simulink library "tqr"  (R2021b)
settings: Solver=VariableStepAuto  StartTime=0.0  StopTime=10.0  RelTol=1e-3
undefined symbols (not defined in the file or in its folder): ATQR_AltRDCActiveFEDUInc_X_pct, ATQR_AltRDCActiveFEDUInc_Y_enum, ATQR_AltRDCActiveFEDUTs_X_pct, ATQR_AltRDCActiveFEDUTs_Y_enum, ATQR_AltRDCActiveREDUInc_X_pct, ATQR_AltRDCActiveREDUInc_Y_enum, ATQR_AltRDCActiveREDUTs_X_pct, ATQR_AltRDCActiveREDUTs_Y_enum, ATQR_CreepFEDUTqIncSR_X_rpm, ATQR_CreepFEDUTqIncSR_Y_Nm, ATQR_CreepFEDUTs_X_rpm, ATQR_CreepFEDUTs_Y_Nm, ATQR_EcoTqFrIncGain_X_Nm, ATQR_EcoTqFrIncGain_Y_pct, ATQR_EcoTqRrIncGain_X_Nm, ATQR_EcoTqRrIncGain_Y_pct, ATQR_EL1FEDUTqDecSR_Y_Nm, ATQR_EL1FEDUTqIncSR_X_rpm, ATQR_EL1FEDUTqIncSR_Y_pct, ATQR_EL1FEDUTs_X_rpm, ATQR_EL1FEDUTs_Y_Nm, ATQR_EL1REDUTqDecSR_Y_Nm, ATQR_EL1REDUTs_Y_Nm, ATQR_FEDUEL1RegenTs_X_rpm, ATQR_FEDUTIPOutTs_X_rpm, ATQR_FrNegRateLimitIncN_X_rpm, ATQR_FrNegRateLimitIncN_Y_Nm, ATQR_FrPosRateLimitIncN_X_rpm, ATQR_FrPosRateLimitIncN_Y_Nm, ATQR_FShaftSpdTqLimCoe_X_rpm, ATQR_FTimerTqLimCoe_X_s, ATQR_FTqZeroTransUpBoundN_X_rpm, ATQR_NL1FEDUTqDecSR_Y_Nm, ATQR_NL1FEDUTqIncSR_X_rpm, ATQR_NL1FEDUTqIncSR_Y_pct, ATQR_NL1FEDUTs_X_rpm, ATQR_NL1FEDUTs_Y_Nm, ATQR_NL1REDUTqDecSR_Y_Nm, ATQR_NL1REDUTs_Y_Nm, ATQR_NormalTqFrIncGain_X_Nm, ATQR_NormalTqFrIncGain_Y_pct, ATQR_NormalTqRrIncGain_X_Nm, ATQR_NormalTqRrIncGain_Y_pct, ATQR_RrNegRateLimitIncN_X_rpm, ATQR_RrNegRateLimitIncN_Y_Nm, ATQR_RrPosRateLimitIncN_X_rpm, ATQR_RrPosRateLimitIncN_Y_Nm, ATQR_RShaftSpdTqLimCoe_X_rpm, ATQR_RTimerTqLimCoe_X_s, ATQR_SL1FEDUTqDecSR_Y_Nm, ATQR_SL1FEDUTqIncSR_X_rpm, ATQR_SL1FEDUTqIncSR_Y_pct, ATQR_SL1FEDUTs_X_rpm, ATQR_SL1FEDUTs_Y_Nm, ATQR_SL1REDUTqDecSR_Y_Nm, ATQR_SL1REDUTs_Y_Nm, ATQR_SportTqFrIncGain_X_Nm, ATQR_SportTqFrIncGain_Y_pct, ATQR_SportTqRrIncGain_X_Nm, ATQR_SportTqRrIncGain_Y_pct ... (+287)
libraries: hcu_lib x19, simulink x17, $bdroot x3
(part 5 of 10)

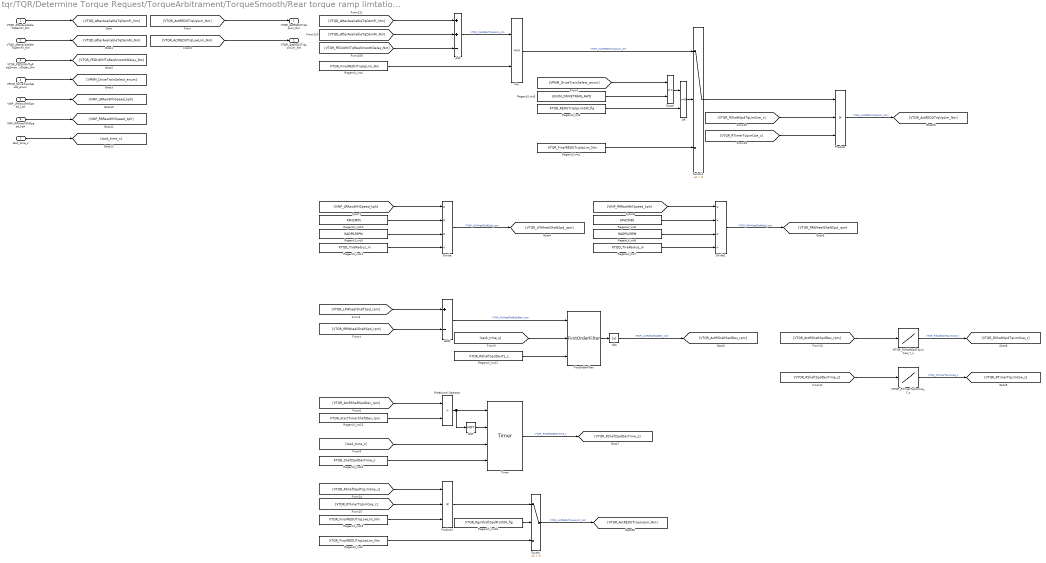
== system tqr/TQR/Determine Torque Request/TorqueArbitrament/TorqueSmooth/Rear torque ramp limtation and determination ==
  VTQD_AfterAvailableTqDemFr_Nm : Inport
  VTQD_AfterAvailableTqDemRr_Nm : Inport  Port=2
  VTQR_FEDUWhlTqReqSmoothDelay_Nm : Inport  Port=3
  VPMM_DriveTrainSelect_enum : Inport  Port=4
  VINP_LRRawWhlSpeed_kph : Inport  Port=5
  VINP_RRRawWhlSpeed_kph : Inport  Port=6
  task_time_s : Inport  Port=7
  Abs : Abs
  Add : Sum  Inputs=++-
  Add1 : Sum  Inputs=+-
  Divide : Product  Inputs=***/
  Divide1 : Product  Inputs=***/
  Equal : RelationalOperator  Operator===  OutDataTypeStr=boolean  RndMeth=Simplest
  FirstOrderFilter : hcu_lib/Basic_Blocks/FirstOrderFilter
  MTQR_RShaftSpdTqLimCoe_Y_c : Lookup_n-D  NumberOfTableDimensions=1  BreakpointsForDimension1=ATQR_RShaftSpdTqLimCoe_X_rpm  Table=MTQR_RShaftSpdTqLimCoe_Y_c  InternalRulePriority=Speed  RndMeth=Simplest  InputSameDT=on
  MTQR_RTimerTqLimCoe_Y_c : Lookup_n-D  NumberOfTableDimensions=1  BreakpointsForDimension1=ATQR_RTimerTqLimCoe_X_s  Table=MTQR_RTimerTqLimCoe_Y_c  InternalRulePriority=Speed  RndMeth=Simplest  InputSameDT=on
  Min : MinMax  Inputs=2
  NOT : Logic  Operator=NOT  AllPortsSameDT=off  OutDataTypeStr=boolean
  OR : Logic  AllPortsSameDT=off  OutDataTypeStr=boolean
  Product : Product  Inputs=3
  Product1 : Product  Inputs=3
  RegenLV_inc1 : Constant  Value=KTQR_FinalREDUTrqUpLim_Nm  OutDataTypeStr=single
  RegenLV_inc10 : Constant  Value=KPH2MPS  OutDataTypeStr=single
  RegenLV_inc11 : Constant  Value=KTQD_TireRadius_m  OutDataTypeStr=single
  RegenLV_inc12 : Constant  Value=KTQR_RShaftSpdDevTs_c  OutDataTypeStr=single
  RegenLV_inc13 : Constant  Value=KTQR_StartTimerShaftDev_rpm  OutDataTypeStr=single
  RegenLV_inc14 : Constant  Value=KTQR_ShaftSpdDevTime_s  OutDataTypeStr=single
  RegenLV_inc15 : Constant  Value=KTQR_FinalREDUTrqLowLim_Nm  OutDataTypeStr=single
  RegenLV_inc16 : Constant  Value=KTQR_RgnShaftSpdProtSW_flg  OutDataTypeStr=single
  RegenLV_inc2 : Constant  Value=KTQR_FinalREDUTrqLowLim_Nm  OutDataTypeStr=single
  RegenLV_inc3 : Constant  Value=KTQR_REDUTrqUpLimSW_flg  OutDataTypeStr=single
  RegenLV_inc4 : Constant  Value=KTQR_FinalREDUTrqUpLim_Nm  OutDataTypeStr=single
  RegenLV_inc5 : Constant  Value=ENUM_DRIVETRAIN_AWD  OutDataTypeStr=single
  RegenLV_inc6 : Constant  Value=KPH2MPS  OutDataTypeStr=single
  RegenLV_inc7 : Constant  Value=KTQD_TireRadius_m  OutDataTypeStr=single
  RegenLV_inc8 : Constant  Value=RADPS2RPM  OutDataTypeStr=single
  RegenLV_inc9 : Constant  Value=RADPS2RPM  OutDataTypeStr=single
  Relational Operator : RelationalOperator  Operator=>  OutDataTypeStr=boolean  RndMeth=Simplest
  Switch : Switch  Criteria=u2 > Threshold
  Switch1 : Switch  Criteria=u2 > Threshold
  Timer : hcu_lib/Basic_Blocks/Timer
  VTQR_ActREDUTrqUpLim_Nm : Outport
  VTQR_ActREDUTrqLowLim_Nm : Outport  Port=2
  wires:
  Add/1 -> Min/1  "VTQR_CalREDUTrqUpLim_Nm"
  RegenLV_inc4/1 -> Min/2
  [VTQR_FEDUWhlTqReqSmoothDelay_Nm] -> Add/3
  Min/1 -> Switch1/1  "VTQR_CoorREDUTrqUpLim_Nm"
  [VTQD_AfterAvailableTqDemFr_Nm] -> Add/1
  [VTQD_AfterAvailableTqDemRr_Nm] -> Add/2
  RegenLV_inc1/1 -> Switch1/3
  VTQD_AfterAvailableTqDemFr_Nm/1 -> [VTQD_AfterAvailableTqDemFr_Nm]
  VTQD_AfterAvailableTqDemRr_Nm/1 -> [VTQD_AfterAvailableTqDemRr_Nm]
  VTQR_FEDUWhlTqReqSmoothDelay_Nm/1 -> [VTQR_FEDUWhlTqReqSmoothDelay_Nm]
  VPMM_DriveTrainSelect_enum/1 -> [VPMM_DriveTrainSelect_enum]
  [VTQR_ActREDUTrqUpLim_Nm] -> VTQR_ActREDUTrqUpLim_Nm/1
  [VTQR_ActREDUTrqLowLim_Nm] -> VTQR_ActREDUTrqLowLim_Nm/1
  OR/1 -> Switch1/2
  Equal/1 -> OR/1
  RegenLV_inc5/1 -> Equal/2
  [VPMM_DriveTrainSelect_enum] -> Equal/1
  RegenLV_inc3/1 -> OR/2
  RegenLV_inc10/1 -> Divide/2
  RegenLV_inc9/1 -> Divide/3
  RegenLV_inc11/1 -> Divide/4
  Divide/1 -> [VTQR_LFWheelShaftSpd_rpm]  "VTQR_LRWheelShaftSpd_rpm"
  Divide1/1 -> [VTQR_RRWheelShaftSpd_rpm]  "VTQR_RRWheelShaftSpd_rpm"
  RegenLV_inc7/1 -> Divide1/4
  RegenLV_inc8/1 -> Divide1/3
  RegenLV_inc6/1 -> Divide1/2
  [VINP_RRRawWhlSpeed_kph] -> Divide1/1
  Add1/1 -> FirstOrderFilter/1  "VTQR_RWheelShaftSpdDev_rpm"
  [task_time_s] -> FirstOrderFilter/2
  [VTQR_RRWheelShaftSpd_rpm] -> Add1/2
  RegenLV_inc12/1 -> FirstOrderFilter/3
  FirstOrderFilter/1 -> Abs/1
  Abs/1 -> [VTQR_ActRShaftSpdDev_rpm]  "VTQR_ActRShaftSpdDev_rpm"
  [VTQR_ActRShaftSpdDev_rpm] -> Relational Operator/1
  [VTQR_LFWheelShaftSpd_rpm] -> Add1/1
  RegenLV_inc13/1 -> Relational Operator/2
  Relational Operator/1 -> Timer/1, NOT/1
  NOT/1 -> Timer/2
  [task_time_s] -> Timer/3
  RegenLV_inc14/1 -> Timer/4
  Timer/1 -> [VTQR_RShaftSpdDevTime_s]  "VTQR_RShaftSpdDevTime_s"
  [VTQR_ActRShaftSpdDev_rpm] -> MTQR_RShaftSpdTqLimCoe_Y_c/1
  MTQR_RShaftSpdTqLimCoe_Y_c/1 -> [VTQR_RShaftSpdTqLimCoe_c]  "VTQR_RShaftSpdTqLimCoe_c"
  MTQR_RTimerTqLimCoe_Y_c/1 -> [VTQR_RTimerTqLimCoe_c]  "VTQR_RTimerTqLimCoe_c"
  [VTQR_RShaftSpdDevTime_s] -> MTQR_RTimerTqLimCoe_Y_c/1
  Product/1 -> [VTQR_ActREDUTrqUpLim_Nm]  "VTQR_ActREDUTrqUpLim_Nm"
  Switch1/1 -> Product/1
  [VTQR_RShaftSpdTqLimCoe_c] -> Product/2
  [VTQR_RTimerTqLimCoe_c] -> Product/3
  task_time_s/1 -> [task_time_s]
  VINP_RRRawWhlSpeed_kph/1 -> [VINP_RRRawWhlSpeed_kph]
  VINP_LRRawWhlSpeed_kph/1 -> [VINP_LRRawWhlSpeed_kph]
  [VINP_LRRawWhlSpeed_kph] -> Divide/1
  Switch/1 -> [VTQR_ActREDUTrqLowLim_Nm]  "VTQR_ActREDUTrqLowLim_Nm"
  RegenLV_inc2/1 -> Switch/3
  Product1/1 -> Switch/1
  RegenLV_inc15/1 -> Product1/3
  [VTQR_RTimerTqLimCoe_c] -> Product1/2
  [VTQR_RShaftSpdTqLimCoe_c] -> Product1/1
  RegenLV_inc16/1 -> Switch/2

== system tqr/TQR/Determine Torque Request/TorqueArbitrament/TorqueSmooth/Rear wheel first order filter input torque command determination ==
  VTQR_RrTqZeroTrans_enum : Inport
  VTQR_RrTqZeroTransUpBound_Nm : Inport  Port=2
  VTQR_RrTqZeroTransLowBound_Nm : Inport  Port=3
  VTQD_AfterAvailableTqDemRr_Nm : Inport  Port=4
  VTQR_RrFirstOrderOutTqDelay_Nm : Inport  Port=5
  VTQR_RrGearChange_flg : Inport  Port=6
  VTQR_RampTqCMDGain_c : Inport  Port=7
  AND : Logic  AllPortsSameDT=off  OutDataTypeStr=boolean
  Constant1 : Constant  Value=ZERO_FLOAT
  Constant2 : Constant  Value=KTQR_GearChangeTqSW_flg
  Constant3 : Constant  Value=ENUM_TQZEROTRANS_NOZEROTRANS
  Constant4 : Constant  Value=KTQR_NewRampArchSW_flg
  Constant5 : Constant  Value=ONE_FLOAT
  Product : Product
  Relational Operator : RelationalOperator  Operator===  OutDataTypeStr=boolean  RndMeth=Simplest
  Relational Operator1 : RelationalOperator  OutDataTypeStr=boolean  RndMeth=Simplest
  Relational Operator2 : RelationalOperator  Operator=<=  OutDataTypeStr=boolean  RndMeth=Simplest
  Switch : Switch  Criteria=u2 ~= 0
  Switch1 : Switch  Criteria=u2 ~= 0
  Switch2 : Switch  Criteria=u2 ~= 0
  Switch3 : Switch  Criteria=u2 > Threshold
  Switch4 : Switch  Criteria=u2 > Threshold
  VTQR_RrFirstOrderInpTq_Nm : Outport
  wires:
  Switch3/1 -> VTQR_RrFirstOrderInpTq_Nm/1  "VTQR_RrFirstOrderInpTq_Nm"
  [VTQR_RrTqZeroTransUpBound_Nm] -> Switch1/1
  [VTQR_RrTqZeroTransUpBound_Nm] -> Relational Operator1/2
  [VTQR_RrFirstOrderOutTqDelay_Nm] -> Relational Operator1/1
  Relational Operator1/1 -> Switch1/2
  Switch1/1 -> Switch/3
  Relational Operator/1 -> Switch/2
  Constant3/1 -> Relational Operator/2
  [VTQR_RrTqZeroTrans_enum] -> Relational Operator/1
  Relational Operator2/1 -> Switch2/2
  [VTQR_RrActRampTqDem_Nm] -> Switch2/3
  [VTQR_RrTqZeroTransLowBound_Nm] -> Switch2/1
  [VTQR_RrFirstOrderOutTqDelay_Nm] -> Relational Operator2/1
  [VTQR_RrTqZeroTransLowBound_Nm] -> Relational Operator2/2
  Switch2/1 -> Switch1/3
  VTQR_RrTqZeroTransUpBound_Nm/1 -> [VTQR_RrTqZeroTransUpBound_Nm]
  VTQR_RrTqZeroTransLowBound_Nm/1 -> [VTQR_RrTqZeroTransLowBound_Nm]
  VTQR_RrFirstOrderOutTqDelay_Nm/1 -> [VTQR_RrFirstOrderOutTqDelay_Nm]
  VTQR_RrGearChange_flg/1 -> [VTQR_RrGearChange_flg]
  VTQR_RrTqZeroTrans_enum/1 -> [VTQR_RrTqZeroTrans_enum]
  VTQD_AfterAvailableTqDemRr_Nm/1 -> [VTQD_AfterAvailableTqDemRr_Nm]
  Constant2/1 -> AND/2
  Constant1/1 -> Switch3/1
  [VTQR_RrGearChange_flg] -> AND/1
  AND/1 -> Switch3/2
  Switch/1 -> Switch3/3
  VTQR_RampTqCMDGain_c/1 -> [VTQR_RampTqCMDGain_c]
  Product/1 -> [VTQR_RrActRampTqDem_Nm]  "VTQR_RrActRampTqDem_Nm"
  Constant4/1 -> Switch4/2
  Switch4/1 -> Product/2
  Constant5/1 -> Switch4/3
  [VTQR_RampTqCMDGain_c] -> Switch4/1
  [VTQR_RrActRampTqDem_Nm] -> Switch/1
  [VTQD_AfterAvailableTqDemRr_Nm] -> Product/1

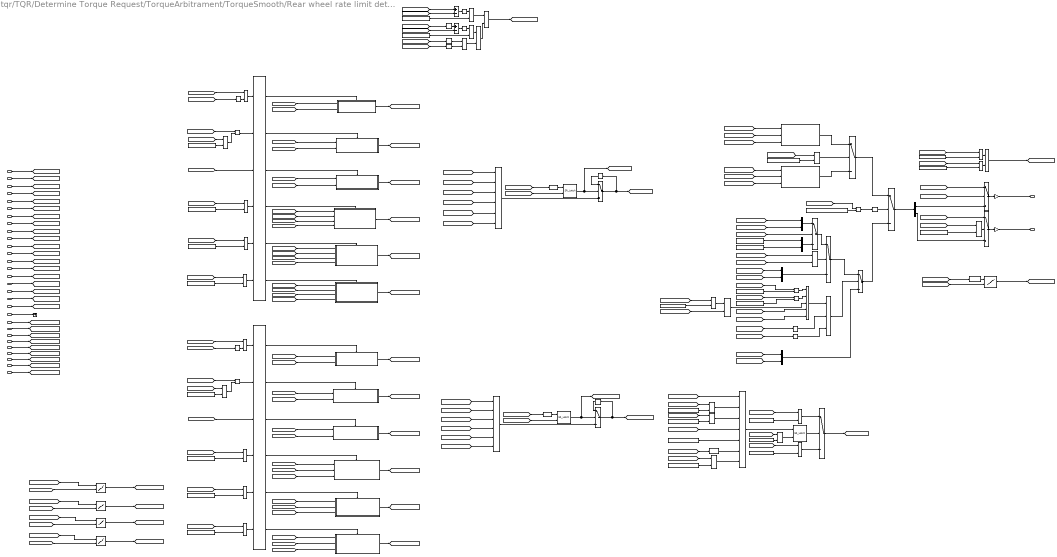
== system tqr/TQR/Determine Torque Request/TorqueArbitrament/TorqueSmooth/Rear wheel rate limit determination ==
  VTQR_RrTqZeroTrans_enum : Inport
  VTQD_TqSourceRr_enum : Inport  Port=2
  VTQD_TqTargetShaftSpd_rpm : Inport  Port=3
  VTQD_LimpHomeAct_flg : Inport  Port=4
  VTQR_EVDriveMode_enum : Inport  Port=5
  VDHP_ActAPSPosn_pct : Inport  Port=6
  VTQR_REDUWhlTqReqSmoothDelay_Nm : Inport  Port=7
  VTQD_EVDriveModeValid_flg : Inport  Port=8
  VTQD_RegenMode_enum : Inport  Port=9
  VVMC_ACCPedalOvrd_flg : Inport  Port=10
  VVMC_CCPedalOvrd_flg : Inport  Port=11
  VTQD_CreepPrLoadEnable_flg : Inport  Port=12
  VTQD_RegenTqLimitEn_flg : Inport  Port=13
  VTQD_RDCActive_enum : Inport  Port=14
  VTQD_PreLoadPreEn_flg : Inport  Port=15
  VTQR_NoABSREDUWhlTqReq_Nm : Inport  Port=16
  VTQR_RampREDUWhlTqReq_Nm : Inport  Port=17
  VTQR_RrFirstOrderInpTq_Nm : Inport  Port=18
  VVMC_ActMaxSlideRate_pct : Inport  Port=19
  VTQD_PedAccTqEn_flg : Inport  Port=20
  VVMC_MSAWhlTqActive_flg : Inport  Port=21
  VINP_ACCVehHoldReq_flg : Inport  Port=22
  VINP_GRADE_Deg : Inport  Port=23
  VTQD_VehActSpd_kph : Inport  Port=24
  VVMC_ADASActive_flg : Inport  Port=25
  VPMM_DriveTrainSelect_enum : Inport  Port=26
  VINP_RrPTCSActive_flg : Inport  Port=27
  VINP_IVISnowModeCmd_flg : Inport  Port=28
  VINP_VehicleType_enum : Inport  Port=29
  AND{,2..4} (4 alike) : Logic  AllPortsSameDT=off  OutDataTypeStr=boolean
  AND1 : Logic  Inputs=3  AllPortsSameDT=off  OutDataTypeStr=boolean
  AND5 : Logic  Inputs=7  AllPortsSameDT=off  OutDataTypeStr=boolean
  Abs : Abs
  Abs4 : Abs
  Add : Sum  Inputs=+-
  Add1 : Sum  Inputs=+-
  Constant : Constant  Value=KTQR_ACCHoldPdovrdGrade_Deg
  Constant1 : Constant  Value=ENUM_TQZEROTRANS_NOZEROTRANS
  Constant10 : Constant  Value=ENUM_TQSOURCE_MSA
  Constant11 : Constant  Value=KTQR_ACCHoldPdovrdVeh_kph
  Constant12 : Constant  Value=KTQR_ARegenLatchEnTq_Nm
  Constant13 : Constant  Value=KTQR_ACCHoldPdovrdSW_flg
  Constant14 : Constant  Value=ENUM_DRIVETRAIN_RWD
  Constant15 : Constant  Value=KTQR_ACCHoldPdovrdInc_Nm
  Constant16 : Constant  Value=KTQR_ACCHoldPdovrdInc_Nm
  Constant17 : Constant  Value=ZERO_FLOAT
  Constant18 : Constant  Value=ENUM_VEHICLETYPE_D31L24
  Constant19 : Constant  Value=ENUM_VEHICLETYPE_D31L24
  Constant2 : Constant  Value=KTQR_DriveModeChangeTq_Nm
  Constant22 : Constant  Value=ENUM_DRIVEMODE_ECO
  Constant23 : Constant  Value=ENUM_DRIVEMODE_NRM
  Constant24 : Constant  Value=ENUM_DRIVEMODE_SPORT
  Constant26 : Constant  Value=ENUM_DRIVEMODE_ECO
  Constant27 : Constant  Value=ENUM_DRIVEMODE_NRM
  Constant28 : Constant  Value=ENUM_DRIVEMODE_SPORT
  Constant3 : Constant  Value=ENUM_TQSOURCE_CC
  Constant34 : Constant  Value=ENUM_TQSOURCE_ADAS
  Constant4 : Constant  Value=ENUM_TQZEROTRANS_POSITIVE
  Constant5 : Constant  Value=ENUM_RDCACTSTA_NOREQUEST
  Constant6 : Constant  Value=KTQR_RegenTqLimitDecSW_flg
  Constant7 : Constant  Value=KTQR_PreLoadTqIncSR_Nm
  Constant8 : Constant  Value=KTQR_DriveModeCMDTqDev_Nm
  Constant9 : Constant  Value=KTQR_PreLoadTqDecSR_Nm
  Data Type Conversion : DataTypeConversion  OutDataTypeStr=single
  Delay{,1..4} (5 alike) : Delay  DelayLength=1
  Demux : Demux  Outputs=2
  Detect Change : simulink/Logic and Bit Operations/Detect Change  vinit=0  OutDataTypeStr=boolean
  Detect Change1 : simulink/Logic and Bit Operations/Detect Change  vinit=0  OutDataTypeStr=boolean
  Detect Increase : simulink/Logic and Bit Operations/Detect Increase  vinit=0.0  OutDataTypeStr=boolean
  Equal : RelationalOperator  OutDataTypeStr=boolean  RndMeth=Simplest
  Equal1 : RelationalOperator  Operator=<=  OutDataTypeStr=boolean  RndMeth=Simplest
  Equal2 : RelationalOperator  Operator=~=  OutDataTypeStr=boolean  RndMeth=Simplest
  Equal{3,20..21,23..25,27} (7 alike) : RelationalOperator  Operator===  OutDataTypeStr=boolean  RndMeth=Simplest
  Equal4 : RelationalOperator  OutDataTypeStr=boolean  RndMeth=Simplest
  Equal5 : RelationalOperator  Operator=~=  OutDataTypeStr=boolean  RndMeth=Simplest
  Equal6 : RelationalOperator  Operator=~=  OutDataTypeStr=boolean  RndMeth=Simplest
  Gain : Gain
  Gain1 : Gain
  If : If  NumInputs=6  IfExpression=u1~= 0  ElseIfExpressions=u2 ~= 0, u3 ~= 0,u4 ~= 0,u5 ~= 0
  If1 : If  NumInputs=6  IfExpression=u1~= 0  ElseIfExpressions=u2 ~= 0, u3 ~= 0,u4 ~= 0,u5 ~= 0
  Logical Operator : Logic  AllPortsSameDT=off  OutDataTypeStr=boolean
  Logical Operator1 : Logic  AllPortsSameDT=off  OutDataTypeStr=boolean
  Logical Operator10 : Logic  Operator=OR  AllPortsSameDT=off  OutDataTypeStr=boolean
  Logical Operator11 : Logic  Operator=NOT  AllPortsSameDT=off  OutDataTypeStr=boolean
  Logical Operator12 : Logic  Operator=OR  AllPortsSameDT=off  OutDataTypeStr=boolean
  Logical Operator13 : Logic  Operator=NOT  AllPortsSameDT=off  OutDataTypeStr=boolean
  Logical Operator14 : Logic  Operator=OR  Inputs=5  AllPortsSameDT=off  OutDataTypeStr=boolean
  Logical Operator7 : Logic  Operator=NOT  AllPortsSameDT=off  OutDataTypeStr=boolean
  MTQR_AltRDCActiveREDUInc_Z_Nm : Lookup_n-D  BreakpointsForDimension1=ATQR_AltRDCActiveREDUInc_Y_enum  BreakpointsForDimension2=ATQR_AltRDCActiveREDUInc_X_pct  Table=MTQR_AltRDCActiveREDUInc_Z_Nm  TableDataTypeStr=Inherit: Inherit from 'Table data'  ExtrapMethod=Clip  InternalRulePriority=Speed  RndMeth=Simplest  InputSameDT=on
      settings: InputPortMap=u0,u1
  MTQR_CreepREDUTqDecSR_Z_Nm : Lookup_n-D  BreakpointsForDimension1=ATQR_CreepFEDUTqIncSR_Y_Nm  BreakpointsForDimension2=ATQR_CreepFEDUTqIncSR_X_rpm  Table=MTQR_CreepREDUTqDecSR_Z_Nm  ExtrapMethod=Clip  InternalRulePriority=Speed  RndMeth=Simplest  InputSameDT=on
      settings: InputPortMap=u0,u1
  MTQR_CreepREDUTqIncSR_Z_Nm : Lookup_n-D  BreakpointsForDimension1=ATQR_CreepFEDUTqIncSR_Y_Nm  BreakpointsForDimension2=ATQR_CreepFEDUTqIncSR_X_rpm  Table=MTQR_CreepREDUTqIncSR_Z_Nm  ExtrapMethod=Clip  InternalRulePriority=Speed  RndMeth=Simplest  InputSameDT=on
      settings: InputPortMap=u0,u1
  MTQR_VMCREDUTqDecSR_Z_Nm : Lookup_n-D  BreakpointsForDimension1=ATQR_VMCREDUTqIncSR_Y_Nm  BreakpointsForDimension2=ATQR_VMCFEDUTqIncSR_X_rpm  Table=MTQR_VMCREDUTqDecSR_Z_Nm  ExtrapMethod=Clip  InternalRulePriority=Speed  RndMeth=Simplest  InputSameDT=on
      settings: InputPortMap=u0,u1
  MTQR_VMCREDUTqIncSR_Z_Nm : Lookup_n-D  BreakpointsForDimension1=ATQR_VMCREDUTqIncSR_Y_Nm  BreakpointsForDimension2=ATQR_VMCFEDUTqIncSR_X_rpm  Table=MTQR_VMCREDUTqIncSR_Z_Nm  ExtrapMethod=Clip  InternalRulePriority=Speed  RndMeth=Simplest  InputSameDT=on
      settings: InputPortMap=u0,u1
  Max : MinMax  Function=max  Inputs=2
  Max1 : MinMax  Function=max  Inputs=2
  Merge4 : Merge  Inputs=6
  Merge5 : Merge  Inputs=6
  Mux{1..4} (4 alike) : Mux  Inputs=2
  NOT : Logic  Operator=NOT  AllPortsSameDT=off  OutDataTypeStr=boolean
  NOT1 : Logic  Operator=NOT  AllPortsSameDT=off  OutDataTypeStr=boolean
  Negative Rate limit Determination : Subsystem  TreatAsAtomicUnit=on
  OR : Logic  Operator=OR  AllPortsSameDT=off  OutDataTypeStr=boolean
  OR2 : Logic  Operator=OR  AllPortsSameDT=off  OutDataTypeStr=boolean
  OR3 : Logic  Operator=OR  AllPortsSameDT=off  OutDataTypeStr=boolean
  Positive Rate limit Determination : Subsystem  TreatAsAtomicUnit=on
  Relational Operator{,1,3..4,7} (5 alike) : RelationalOperator  Operator===  OutDataTypeStr=boolean  RndMeth=Simplest
  Relational Operator2 : RelationalOperator  Operator=<=  OutDataTypeStr=boolean  RndMeth=Simplest
  Relational Operator5 : RelationalOperator  Operator=<  OutDataTypeStr=boolean  RndMeth=Simplest
  Relational Operator6 : RelationalOperator  OutDataTypeStr=boolean  RndMeth=Simplest
  SR_Latch1 : hcu_lib/Basic_Blocks/SR_Latch
  SR_Latch2 : hcu_lib/Basic_Blocks/SR_Latch
  SR_Latch3 : hcu_lib/Basic_Blocks/SR_Latch
  Switch{,4..7} (5 alike) : Switch  Criteria=u2 > Threshold
  Switch1 : Switch  Criteria=u2 ~= 0  Threshold=0.5
  Switch13 : Switch  Criteria=u2 ~= 0
  Switch2 : Switch  Criteria=u2 ~= 0
  Switch3 : Switch  Criteria=u2 ~= 0  Threshold=0.5
  Switch8 : Switch  Criteria=u2 ~= 0
  Terminator : Terminator
  VTQR_ECOREDURateLimitDec_Nm : Subsystem  AncestorBlock=tqr/TQR/Determine Torque Request/TorqueArbitrament/TorqueSmooth/Front wheel rate limit determination/VTQR_ECOFEDURateLimitDec_Nm  TreatAsAtomicUnit=on
  VTQR_ECOREDURateLimitInc_Nm : Subsystem  TreatAsAtomicUnit=on
  VTQR_LHMREDURateLimitDec_Nm : Subsystem  AncestorBlock=tqr/TQR/Determine Torque Request/TorqueArbitrament/TorqueSmooth/VTQR_LHMREDURateLimitDec_Nm  TreatAsAtomicUnit=on
  VTQR_LHMREDURateLimitInc_Nm : Subsystem  TreatAsAtomicUnit=on
  VTQR_NORMALREDURateLimitDec_Nm : Subsystem  AncestorBlock=tqr/TQR/Determine Torque Request/TorqueArbitrament/TorqueSmooth/Rear wheel rate limit determination/VTQR_ECOFEDURateLimitDec_Nm  TreatAsAtomicUnit=on
  VTQR_NORMALREDURateLimitInc_Nm : Subsystem  TreatAsAtomicUnit=on
  VTQR_SNOWREDURateLimitDec_Nm : Subsystem  TreatAsAtomicUnit=on
  VTQR_SNOWREDURateLimitInc_Nm : Subsystem  TreatAsAtomicUnit=on
  VTQR_SPORTREDURateLimitDec_Nm : Subsystem  AncestorBlock=tqr/TQR/Determine Torque Request/TorqueArbitrament/TorqueSmooth/Rear wheel rate limit determination/VTQR_ECOFEDURateLimitDec_Nm  TreatAsAtomicUnit=on
  VTQR_SPORTREDURateLimitInc_Nm : Subsystem  TreatAsAtomicUnit=on
  VTQR_TCSREDURateLimitDec_Nm : Subsystem  TreatAsAtomicUnit=on
  VTQR_TCSREDURateLimitInc_Nm : Subsystem  TreatAsAtomicUnit=on
  VTQR_RrRateLimitInc_Nm : Outport
  VTQR_RrRateLimitDec_Nm : Outport  Port=2
  wires:
  VTQD_TqTargetShaftSpd_rpm/1 -> [VTQD_TqTargetShaftSpd_rpm]
  Gain1/1 -> VTQR_RrRateLimitDec_Nm/1  "VTQR_RrRateLimitDec_Nm"
  Gain/1 -> VTQR_RrRateLimitInc_Nm/1  "VTQR_RrRateLimitInc_Nm"
  [VTQR_REDURateLimitDec_Nm] -> Mux4/2
  [VTQR_REDURateLimitInc_Nm] -> Mux4/1
  [VTQR_VMCREDUTqDecSR_Nm] -> Mux3/2
  [VTQR_VMCREDUTqIncSR_Nm] -> Mux3/1
  Positive Rate limit Determination/1(VTQR_PosRateLimit_mux) -> Switch1/1
  Negative Rate limit Determination/1(VTQR_NegRateLimit_mux) -> Switch1/3
  Switch3/1 -> Demux/1
  Switch1/1 -> Switch3/1
  Constant4/1 -> Relational Operator1/2
  Relational Operator1/1 -> Switch1/2
  [VTQR_RrTqZeroTrans_enum] -> Relational Operator1/1
  [VTQR_RrTqZeroTrans_enum] -> Relational Operator/1
  Constant1/1 -> Relational Operator/2
  Relational Operator/1 -> Logical Operator7/1
  Logical Operator7/1 -> Switch3/2
  Switch13/1 -> Switch3/3
  Mux4/1 -> Switch13/3
  AND1/1 -> Switch13/2
  VTQD_TqSourceRr_enum/1 -> [VTQD_TqSourceRr_enum]
  VTQR_RrTqZeroTrans_enum/1 -> [VTQR_RrTqZeroTrans_enum]
  MTQR_VMCREDUTqIncSR_Z_Nm/1 -> [VTQR_VMCREDUTqIncSR_Nm]  "VTQR_VMCREDUTqIncSR_Nm"
  Constant27/1 -> Equal25/2
  [VDHP_ActAPSPosn_pct] -> VTQR_LHMREDURateLimitInc_Nm/1(VDHP_ActAPSPosn_pct)
  [VTQD_LimpHomeAct_flg] -> Logical Operator12/1
  Constant22/1 -> Equal20/2
  MTQR_VMCREDUTqDecSR_Z_Nm/1 -> [VTQR_VMCREDUTqDecSR_Nm]  "VTQR_VMCREDUTqDecSR_Nm"
  [VTQR_EVDriveMode_enum] -> Equal27/1
  Constant28/1 -> Equal27/2
  [VTQR_EVDriveMode_enum] -> Equal25/1
  [VTQD_EVDriveModeValid_flg] -> Logical Operator11/1
  Logical Operator10/1 -> If/1
  Constant24/1 -> Equal23/2
  [VTQD_LimpHomeAct_flg] -> Logical Operator10/1
  Logical Operator11/1 -> Logical Operator10/2
  [VTQR_EVDriveMode_enum] -> Equal20/1
  VTQR_LHMREDURateLimitDec_Nm/1(VTQR_LHMREDURateLimitDec_Nm) -> [VTQR_LHMREDURateLimitDec_Nm]
  [VTQR_REDUWhlTqReqSmoothDelay_Nm] -> VTQR_ECOREDURateLimitDec_Nm/1(VTQR_REDUWhlTqReqSmoothDelay_Nm)
  [VTQD_TqTargetShaftSpd_rpm] -> VTQR_NORMALREDURateLimitDec_Nm/2(VTQD_TqTargetShaftSpd_rpm)  "VTQD_TqTargetShaftSpd_rpm"
  [VTQR_REDUWhlTqReqSmoothDelay_Nm] -> VTQR_LHMREDURateLimitDec_Nm/1(VTQR_REDUWhlTqReqSmooth_Nm)
  [VTQD_TqTargetShaftSpd_rpm] -> VTQR_LHMREDURateLimitDec_Nm/2(VTQD_TqTargetShaftSpd_rpm)  "VTQD_TqTargetShaftSpd_rpm"
  [VTQR_REDUWhlTqReqSmoothDelay_Nm] -> VTQR_NORMALREDURateLimitDec_Nm/1(VTQR_REDUWhlTqReqSmoothDelay_Nm)
  [VTQR_REDUWhlTqReqSmoothDelay_Nm] -> VTQR_SPORTREDURateLimitDec_Nm/1(VTQR_REDUWhlTqReqSmoothDelay_Nm)
  [VTQD_TqTargetShaftSpd_rpm] -> VTQR_LHMREDURateLimitInc_Nm/2(VTQD_TqTargetShaftSpd_rpm)  "VTQD_TqTargetShaftSpd_rpm"
  [VTQD_TqTargetShaftSpd_rpm] -> VTQR_ECOREDURateLimitDec_Nm/2(VTQD_TqTargetShaftSpd_rpm)  "VTQD_TqTargetShaftSpd_rpm"
  [VTQD_TqTargetShaftSpd_rpm] -> VTQR_SPORTREDURateLimitDec_Nm/2(VTQD_TqTargetShaftSpd_rpm)  "VTQD_TqTargetShaftSpd_rpm"
  Constant23/1 -> Equal21/2
  [VTQD_EVDriveModeValid_flg] -> Logical Operator13/1
  [VTQR_EVDriveMode_enum] -> Equal23/1
  Logical Operator13/1 -> Logical Operator12/2
  Constant26/1 -> Equal24/2
  [VTQR_EVDriveMode_enum] -> Equal24/1
  [VTQR_EVDriveMode_enum] -> Equal21/1
  VTQD_LimpHomeAct_flg/1 -> [VTQD_LimpHomeAct_flg]
  VTQR_EVDriveMode_enum/1 -> [VTQR_EVDriveMode_enum]
  VDHP_ActAPSPosn_pct/1 -> [VDHP_ActAPSPosn_pct]
  VTQR_REDUWhlTqReqSmoothDelay_Nm/1 -> [VTQR_REDUWhlTqReqSmoothDelay_Nm]
  VTQD_EVDriveModeValid_flg/1 -> [VTQD_EVDriveModeValid_flg]
  Switch/1 -> Gain/1
  VTQD_RegenMode_enum/1 -> [VTQD_RegenMode_enum]
  [VTQD_RegenMode_enum] -> VTQR_NORMALREDURateLimitDec_Nm/3(VTQD_RegenMode_enum)
  [VTQD_RegenMode_enum] -> VTQR_ECOREDURateLimitDec_Nm/3(VTQD_RegenMode_enum)
  [VTQD_RegenMode_enum] -> VTQR_SPORTREDURateLimitDec_Nm/3(VTQD_RegenMode_enum)
  [VTQD_TqTargetShaftSpd_rpm] -> MTQR_VMCREDUTqIncSR_Z_Nm/2
  [VTQR_REDUWhlTqReqSmoothDelay_Nm] -> MTQR_VMCREDUTqIncSR_Z_Nm/1
  [VTQD_TqTargetShaftSpd_rpm] -> MTQR_VMCREDUTqDecSR_Z_Nm/2
  [VTQR_REDUWhlTqReqSmoothDelay_Nm] -> MTQR_VMCREDUTqDecSR_Z_Nm/1
  VVMC_ACCPedalOvrd_flg/1 -> [VVMC_ACCPedalOvrd_flg]
  VVMC_CCPedalOvrd_flg/1 -> [VVMC_CCPedalOvrd_flg]
  [VTQD_TqSourceRr_enum] -> Relational Operator4/1
  [VTQD_TqSourceRr_enum] -> Relational Operator3/1
  Constant3/1 -> Relational Operator3/2
  Constant34/1 -> Relational Operator4/2
  NOT/1 -> AND1/2
  [VVMC_ACCPedalOvrd_flg] -> NOT/1
  [VVMC_CCPedalOvrd_flg] -> NOT1/1
  NOT1/1 -> AND1/3
  Logical Operator14/1 -> AND1/1
  Relational Operator3/1 -> Logical Operator14/1
  Relational Operator4/1 -> Logical Operator14/2
  [VTQD_TqTargetShaftSpd_rpm] -> Positive Rate limit Determination/1(VTQD_TqTargetShaftSpd_rpm)
  [VTQD_TqTargetShaftSpd_rpm] -> Negative Rate limit Determination/1(VTQD_TqTargetShaftSpd_rpm)
  [VTQR_REDUWhlTqReqSmoothDelay_Nm] -> Positive Rate limit Determination/2(VTQR_REDUWhlTqReqSmoothDelay_Nm)
  [VTQR_EVDriveMode_enum] -> Positive Rate limit Determination/3(VTQR_EVDriveMode_enum)
  [VTQR_REDUWhlTqReqSmoothDelay_Nm] -> Negative Rate limit Determination/2(VTQR_REDUWhlTqReqSmoothDelay_Nm)
  [VTQR_EVDriveMode_enum] -> Negative Rate limit Determination/3(VTQR_EVDriveMode_enum)
  MTQR_CreepREDUTqDecSR_Z_Nm/1 -> [VTQR_CreepREDUTqDecSR_Nm]  "VTQR_CreepREDUTqDecSR_Nm"
  [VTQD_TqTargetShaftSpd_rpm] -> MTQR_CreepREDUTqDecSR_Z_Nm/2
  [VTQD_TqTargetShaftSpd_rpm] -> MTQR_CreepREDUTqIncSR_Z_Nm/2
  MTQR_CreepREDUTqIncSR_Z_Nm/1 -> [VTQR_CreepREDUTqIncSR_Nm]  "VTQR_CreepREDUTqIncSR_Nm"
  [VTQR_REDUWhlTqReqSmoothDelay_Nm] -> MTQR_CreepREDUTqIncSR_Z_Nm/1
  [VTQR_REDUWhlTqReqSmoothDelay_Nm] -> MTQR_CreepREDUTqDecSR_Z_Nm/1
  [VTQD_CreepPrLoadEnable_flg] -> Logical Operator14/4
  [VTQD_PreLoadPreEn_flg] -> Logical Operator14/5
  [VTQD_PreLoadPreEn_flg] -> OR/2
  [VTQD_CreepPrLoadEnable_flg] -> OR/1
  [VTQR_CreepREDUTqIncSR_Nm] -> Mux1/1
  OR/1 -> Switch2/2
  [VTQR_CreepREDUTqDecSR_Nm] -> Mux1/2
  Mux3/1 -> Switch2/3
  Switch2/1 -> Switch13/1
  [VTQR_RrRDCActRateLimitInc_flg] -> Switch/2
  Demux/1 -> Switch/3
  VTQD_CreepPrLoadEnable_flg/1 -> [VTQD_CreepPrLoadEnable_flg]
  VTQD_PreLoadPreEn_flg/1 -> [VTQD_PreLoadPreEn_flg]
  VTQD_RDCActive_enum/1 -> [VTQD_RDCActive_enum]
  VTQR_NoABSREDUWhlTqReq_Nm/1 -> [VTQR_NoABSREDUWhlTqReq_Nm]
  VTQR_RampREDUWhlTqReq_Nm/1 -> [VTQR_RampREDUWhlTqReq_Nm]
  AND/1 -> [VTQR_RrRDCActRateLimitInc_flg]  "VTQR_RrRDCActRateLimitInc_flg"
  Constant12/1 -> Relational Operator2/2
  [VTQR_RampREDUWhlTqReq_Nm] -> Relational Operator2/1
  Equal2/1 -> AND/2
  Relational Operator2/1 -> AND/1
  Constant5/1 -> Equal2/2
  [VTQD_RDCActive_enum] -> Equal2/1
  VTQR_RrFirstOrderInpTq_Nm/1 -> [VTQR_RrFirstOrderInpTq_Nm]
  OR3/1 -> AND4/2
  [VTQR_RrDrModIncLatch_flg] -> Delay3/1
  [VTQR_RrFirstOrderInpTq_Nm] -> Add1/2
  AND4/1 -> OR2/2
  Relational Operator6/1 -> AND4/1
  [VTQR_RrDrModDecLatch_flg] -> Delay4/1
  [VTQR_NoABSREDUWhlTqReq_Nm] -> Add/1
  Detect Change/1 -> SR_Latch1/1
  Abs/1 -> Relational Operator5/1
  Constant8/1 -> Relational Operator6/2
  Delay4/1 -> OR3/2
  [VTQR_RrDrModChangeReset_flg] -> SR_Latch1/2
  SR_Latch1/1 -> Switch4/2, [VTQR_RrDrModIncLatch_flg]
  Abs4/1 -> Relational Operator6/1
  OR2/1 -> [VTQR_RrDrModChangeReset_flg]  "VTQR_RrDrModChangeReset_flg"
  Relational Operator5/1 -> OR2/1
  Delay3/1 -> OR3/1
  Delay1/1 -> Add1/1
  Add1/1 -> Abs4/1
  Add/1 -> Abs/1
  [VTQR_RrFirstOrderInpTq_Nm] -> Delay1/1
  Delay/1 -> Switch4/1
  Constant2/1 -> Relational Operator5/2
  Switch4/1 -> Delay/1, [VTQR_OriREDURateLimitInc_Nm]  "VTQR_OriREDURateLimitInc_Nm"
  [VTQR_RrFirstOrderInpTq_Nm] -> Add/2
  [VTQR_EVDriveMode_enum] -> Detect Change/1
  [VTQR_EVDriveMode_enum] -> Detect Change1/1
  [VTQR_RrDrModChangeReset_flg] -> SR_Latch2/2
  SR_Latch2/1 -> Switch5/2, [VTQR_RrDrModDecLatch_flg]
  Switch5/1 -> Delay2/1, [VTQR_REDURateLimitDec_Nm]  "VTQR_REDURateLimitDec_Nm"
  Delay2/1 -> Switch5/1
  Detect Change1/1 -> SR_Latch2/1
  MTQR_AltRDCActiveREDUInc_Z_Nm/1 -> [VTQR_RDCActiveREDUInc_Nm]  "VTQR_RDCActiveREDUInc_Nm"
  Data Type Conversion/1 -> MTQR_AltRDCActiveREDUInc_Z_Nm/1
  [VTQD_RegenMode_enum] -> Data Type Conversion/1
  [VTQR_RDCActiveREDUInc_Nm] -> Switch/1
  [VVMC_ActMaxSlideRate_pct] -> MTQR_AltRDCActiveREDUInc_Z_Nm/2
  VTQD_PedAccTqEn_flg/1 -> Terminator/1
  VTQD_RegenTqLimitEn_flg/1 -> [VTQD_RegenTqLimitEn_flg]
  VVMC_ActMaxSlideRate_pct/1 -> [VVMC_ActMaxSlideRate_pct]
  [VTQR_VMCREDUTqDecSR_Nm] -> Switch7/1
  AND2/1 -> Switch7/2
  Constant6/1 -> AND2/2
  Switch7/1 -> Gain1/1
  Demux/2 -> Switch7/3
  [VTQD_RegenTqLimitEn_flg] -> AND2/1
  [VDHP_ActAPSPosn_pct] -> VTQR_SPORTREDURateLimitInc_Nm/1(VDHP_ActAPSPosn_pct)
  [VTQD_TqTargetShaftSpd_rpm] -> VTQR_ECOREDURateLimitInc_Nm/2(VTQD_TqTargetShaftSpd_rpm)  "VTQD_TqTargetShaftSpd_rpm"
  [VTQD_RegenMode_enum] -> VTQR_ECOREDURateLimitInc_Nm/3(VTQD_RegenMode_enum)
  [VTQD_RegenMode_enum] -> VTQR_NORMALREDURateLimitInc_Nm/3(VTQD_RegenMode_enum)
  [VTQD_RegenMode_enum] -> VTQR_SPORTREDURateLimitInc_Nm/3(VTQD_RegenMode_enum)
  [VTQD_TqTargetShaftSpd_rpm] -> VTQR_NORMALREDURateLimitInc_Nm/2(VTQD_TqTargetShaftSpd_rpm)  "VTQD_TqTargetShaftSpd_rpm"
  [VTQD_TqTargetShaftSpd_rpm] -> VTQR_SPORTREDURateLimitInc_Nm/2(VTQD_TqTargetShaftSpd_rpm)  "VTQD_TqTargetShaftSpd_rpm"
  [VDHP_ActAPSPosn_pct] -> VTQR_ECOREDURateLimitInc_Nm/1(VDHP_ActAPSPosn_pct)
  [VTQR_REDUWhlTqReqSmoothDelay_Nm] -> VTQR_NORMALREDURateLimitInc_Nm/4(VTQR_REDUWhlTqReqSmoothDelay_Nm)
  [VTQR_REDUWhlTqReqSmoothDelay_Nm] -> VTQR_ECOREDURateLimitInc_Nm/4(VTQR_REDUWhlTqReqSmoothDelay_Nm)
  [VTQR_REDUWhlTqReqSmoothDelay_Nm] -> VTQR_SPORTREDURateLimitInc_Nm/4(VTQR_REDUWhlTqReqSmoothDelay_Nm)
  [VDHP_ActAPSPosn_pct] -> VTQR_NORMALREDURateLimitInc_Nm/1(VDHP_ActAPSPosn_pct)
  Switch6/1 -> Switch2/1
  Mux1/1 -> Switch6/1
  [VTQD_CreepPrLoadEnable_flg] -> Switch6/2
  Mux2/1 -> Switch6/3
  Constant7/1 -> Mux2/1
  Constant9/1 -> Mux2/2
  VVMC_MSAWhlTqActive_flg/1 -> [VVMC_MSAWhlTqActive_flg]
  [VTQD_TqSourceRr_enum] -> Relational Operator7/1
  Constant10/1 -> Relational Operator7/2
  Relational Operator7/1 -> AND3/1
  [VVMC_MSAWhlTqActive_flg] -> AND3/2
  AND3/1 -> Logical Operator14/3
  VINP_ACCVehHoldReq_flg/1 -> [VINP_ACCVehHoldReq_flg]
  VINP_GRADE_Deg/1 -> [VINP_GRADE_Deg]
  [VINP_GRADE_Deg] -> Equal/1
  Constant/1 -> Equal/2
  VTQD_VehActSpd_kph/1 -> [VTQD_VehActSpd_kph]
  [VTQD_VehActSpd_kph] -> Equal1/1
  Constant11/1 -> Equal1/2
  VVMC_ADASActive_flg/1 -> [VVMC_ADASActive_flg]
  [VVMC_ACCPedalOvrd_flg] -> AND5/1
  Equal/1 -> AND5/2
  Equal1/1 -> AND5/3
  [VVMC_ADASActive_flg] -> AND5/4
  [VINP_ACCVehHoldReq_flg] -> Detect Increase/1
  Detect Increase/1 -> AND5/6
  Constant13/1 -> AND5/5
  VPMM_DriveTrainSelect_enum/1 -> [VPMM_DriveTrainSelect_enum]
  [VPMM_DriveTrainSelect_enum] -> Equal3/1
  Constant14/1 -> Equal3/2
  Equal3/1 -> AND5/7
  AND5/1 -> SR_Latch3/1  "VTQR_ACCHoldPdovrdInc_flg"
  [VTQR_OriREDURateLimitInc_Nm] -> Equal4/1
  Constant15/1 -> Equal4/2
  Equal4/1 -> SR_Latch3/2
  SR_Latch3/1 -> Switch8/2
  Max/1 -> Switch8/1
  [VTQR_OriREDURateLimitInc_Nm] -> Max/1
  Constant16/1 -> Max/2
  Constant17/1 -> Max1/2
  [VTQR_OriREDURateLimitInc_Nm] -> Max1/1
  Max1/1 -> Switch8/3
  Switch8/1 -> [VTQR_REDURateLimitInc_Nm]  "VTQR_REDURateLimitInc_Nm"
  Equal23/1 -> If/6
  Equal20/1 -> If/5
  Equal21/1 -> If/4
  [VINP_IVISnowModeCmd_flg] -> If/3
  If/6 -> VTQR_SPORTREDURateLimitInc_Nm/Action
  If/5 -> VTQR_ECOREDURateLimitInc_Nm/Action
  If/4 -> VTQR_NORMALREDURateLimitInc_Nm/Action
  [VDHP_ActAPSPosn_pct] -> VTQR_TCSREDURateLimitInc_Nm/1(VDHP_ActAPSPosn_pct)
  [VTQD_TqTargetShaftSpd_rpm] -> VTQR_TCSREDURateLimitInc_Nm/2(VTQD_TqTargetShaftSpd_rpm)
  If/2 -> VTQR_TCSREDURateLimitInc_Nm/Action
  [VTQD_TqTargetShaftSpd_rpm] -> VTQR_SNOWREDURateLimitInc_Nm/2(VTQD_TqTargetShaftSpd_rpm)
  [VDHP_ActAPSPosn_pct] -> VTQR_SNOWREDURateLimitInc_Nm/1(VDHP_ActAPSPosn_pct)
  If/3 -> VTQR_SNOWREDURateLimitInc_Nm/Action
  VTQR_TCSREDURateLimitInc_Nm/1(VTQR_TCSREDURateLimitInc_Nm) -> [VTQR_TCSREDURateLimitInc_Nm]  "VTQR_TCSREDURateLimitInc_Nm"
  VTQR_SNOWREDURateLimitInc_Nm/1(VTQR_SNOWREDURateLimitInc_Nm) -> [VTQR_SNOWREDURateLimitInc_Nm]  "VTQR_SNOWREDURateLimitInc_Nm"
  VTQR_NORMALREDURateLimitInc_Nm/1(VTQR_NORMALREDURateLimitInc_Nm) -> [VTQR_NORMALREDURateLimitInc_Nm]
  VTQR_ECOREDURateLimitInc_Nm/1(VTQR_ECOREDURateLimitInc_Nm) -> [VTQR_ECOREDURateLimitInc_Nm]
  VTQR_SPORTREDURateLimitInc_Nm/1(VTQR_SPORTREDURateLimitInc_Nm) -> [VTQR_SPORTREDURateLimitInc_Nm]
  [VINP_IVISnowModeCmd_flg] -> If1/3
  Logical Operator12/1 -> If1/1
  Equal27/1 -> If1/6
  Equal24/1 -> If1/5
  Equal25/1 -> If1/4
  If1/1 -> VTQR_LHMREDURateLimitDec_Nm/Action
  VTQR_SPORTREDURateLimitDec_Nm/1(VTQR_SPORTREDURateLimitDec_Nm) -> [VTQR_SPORTREDURateLimitDec_Nm]
  If1/6 -> VTQR_SPORTREDURateLimitDec_Nm/Action
  VTQR_ECOREDURateLimitDec_Nm/1(VTQR_ECOREDURateLimitDec_Nm) -> [VTQR_ECOREDURateLimitDec_Nm]
  If1/5 -> VTQR_ECOREDURateLimitDec_Nm/Action
  VTQR_NORMALREDURateLimitDec_Nm/1(VTQR_NORMALREDURateLimitDec_Nm) -> [VTQR_NORMALREDURateLimitDec_Nm]
  If1/4 -> VTQR_NORMALREDURateLimitDec_Nm/Action
  [VTQR_REDUWhlTqReqSmoothDelay_Nm] -> VTQR_TCSREDURateLimitDec_Nm/1(VTQR_REDUWhlTqReqSmoothDelay_Nm)
  [VTQD_TqTargetShaftSpd_rpm] -> VTQR_TCSREDURateLimitDec_Nm/2(VTQD_TqTargetShaftSpd_rpm)
  VTQR_TCSREDURateLimitDec_Nm/1(VTQR_TCSREDURateLimitDec_Nm) -> [VTQR_TCSREDURateLimitDec_Nm]  "VTQR_TCSREDURateLimitDec_Nm"
  If1/2 -> VTQR_TCSREDURateLimitDec_Nm/Action
  [VTQR_REDUWhlTqReqSmoothDelay_Nm] -> VTQR_SNOWREDURateLimitDec_Nm/1(VTQR_REDUWhlTqReqSmoothDelay_Nm)
  [VTQD_TqTargetShaftSpd_rpm] -> VTQR_SNOWREDURateLimitDec_Nm/2(VTQD_TqTargetShaftSpd_rpm)
  If1/3 -> VTQR_SNOWREDURateLimitDec_Nm/Action
  VTQR_LHMREDURateLimitInc_Nm/1(VTQR_LHMREDURateLimitInc_Nm) -> [VTQR_LHMREDURateLimitInc_Nm]
  [VTQR_SPORTREDURateLimitInc_Nm] -> Merge4/6
  [VTQR_ECOREDURateLimitInc_Nm] -> Merge4/5
  [VTQR_NORMALREDURateLimitInc_Nm] -> Merge4/4
  [VTQR_LHMREDURateLimitInc_Nm] -> Merge4/1
  [VTQR_TCSREDURateLimitInc_Nm] -> Merge4/2
  [VTQR_SNOWREDURateLimitInc_Nm] -> Merge4/3
  Merge4/1 -> Switch4/3
  VTQR_SNOWREDURateLimitDec_Nm/1(VTQR_SNOWREDURateLimitDec_Nm) -> [VTQR_SNOWREDURateLimitDec_Nm]  "VTQR_SNOWREDURateLimitDec_Nm"
  [VTQR_LHMREDURateLimitDec_Nm] -> Merge5/1
  [VTQR_TCSREDURateLimitDec_Nm] -> Merge5/2
  [VTQR_NORMALREDURateLimitDec_Nm] -> Merge5/4
  [VTQR_SPORTREDURateLimitDec_Nm] -> Merge5/6
  [VTQR_SNOWREDURateLimitDec_Nm] -> Merge5/3
  [VTQR_ECOREDURateLimitDec_Nm] -> Merge5/5
  Merge5/1 -> Switch5/3
  VINP_IVISnowModeCmd_flg/1 -> [VINP_IVISnowModeCmd_flg]
  VINP_RrPTCSActive_flg/1 -> [VINP_RrPTCSActive_flg]
  [VINP_VehicleType_enum] -> Equal5/1
  Equal5/1 -> Logical Operator/2
  Constant18/1 -> Equal5/2
  [VINP_RrPTCSActive_flg] -> Logical Operator/1
  Logical Operator/1 -> If/2
  [VINP_VehicleType_enum] -> Equal6/1
  Equal6/1 -> Logical Operator1/2
  Constant19/1 -> Equal6/2
  [VINP_RrPTCSActive_flg] -> Logical Operator1/1
  Logical Operator1/1 -> If1/2
  If/1 -> VTQR_LHMREDURateLimitInc_Nm/Action
  VINP_VehicleType_enum/1 -> [VINP_VehicleType_enum]

== system tqr/TQR/Determine Torque Request/TorqueArbitrament/TorqueSmooth/Zero Torque Revert ==
  VTQD_DRTransfer_flg : Inport
  NTQR_TMTqReq_Nm : Inport  Port=2
  VTQR_TMTqReqLimit_Nm : Inport  Port=3
  Add : Sum  Inputs=+-
  Counter : hcu_lib/Basic_Blocks/Counter
      settings: SourceProductName=HCU Relative Block Library
  Detect Decrease : simulink/Logic and Bit Operations/Detect Decrease  vinit=0.0  OutDataTypeStr=uint8
  Detect Increase : simulink/Logic and Bit Operations/Detect Increase  vinit=0.0  OutDataTypeStr=uint8
  Logical Operator : Logic  Operator=OR  AllPortsSameDT=off  OutDataTypeStr=boolean
  RegenLV_inc5 : Constant  Value=KTQR_TqTransTime_cnt  OutDataTypeStr=single
  RegenLV_inc6 : Constant  Value=KTQR_TqTransTimeMax_cnt  OutDataTypeStr=single
  RegenLV_inc7 : Constant  Value=5  OutDataTypeStr=single
  Relational Operator1 : RelationalOperator  Operator=<=  OutDataTypeStr=boolean  RndMeth=Nearest
  Relational Operator2 : RelationalOperator  Operator=<=  OutDataTypeStr=boolean  RndMeth=Nearest
  SR_Latch : hcu_lib/Basic_Blocks/SR_Latch
      settings: SourceProductName=HCU Relative Block Library
  Unit Delay2 : UnitDelay  SampleTime=-1
  VTQR_ZeroTqRecover_flg : Outport
  wires:
  VTQD_DRTransfer_flg/1 -> Detect Decrease/1, Detect Increase/1
  SR_Latch/1 -> Counter/1, VTQR_ZeroTqRecover_flg/1  "VTQR_ZeroTqRecover_flg"
  Unit Delay2/1 -> Counter/2
  Counter/1 -> Relational Operator2/2
  RegenLV_inc5/1 -> Relational Operator2/1
  Relational Operator2/1 -> Unit Delay2/1  "VINP_RegenLVToggle_flg_InProc"
  RegenLV_inc6/1 -> Counter/3
  Detect Decrease/1 -> SR_Latch/1
  Add/1 -> Relational Operator1/1
  RegenLV_inc7/1 -> Relational Operator1/2
  VTQR_TMTqReqLimit_Nm/1 -> Add/1
  NTQR_TMTqReq_Nm/1 -> Add/2
  Logical Operator/1 -> SR_Latch/2
  Relational Operator1/1 -> Logical Operator/2
  Detect Increase/1 -> Logical Operator/1

== system tqr/TQR/Determine Torque Request/TorqueArbitrament/TorqueSmooth/Front First order filter input tau map and determination/VTQR_ECOFEDUTs_c ==
  VTQR_FEDUWhlTqReqSmoothDelay_Nm : Inport
  VTQD_TqTargetShaftSpd_rpm : Inport  Port=2
  VTQD_RegenMode_enum : Inport  Port=3
  VTQD_RollRegenEnable_flg : Inport  Port=4
  Action Port : ActionPort  ActionPortLabel=elseif(u5 ~= 0)
  Constant10 : Constant  Value=ENUM_REGENLEVEL_LV5
  Constant11 : Constant  Value=ENUM_REGENLEVEL_OPD
  Constant6 : Constant  Value=ENUM_REGENLEVEL_LV1
  Constant7 : Constant  Value=ENUM_REGENLEVEL_LV2
  Constant8 : Constant  Value=ENUM_REGENLEVEL_LV3
  Constant9 : Constant  Value=ENUM_REGENLEVEL_LV4
  Equal{,1..5} (6 alike) : RelationalOperator  Operator===  OutDataTypeStr=boolean  RndMeth=Simplest
  If : If  NumInputs=6  IfExpression=u1~= 0  ElseIfExpressions=u2 ~= 0, u3 ~= 0,u4 ~= 0,u5~=0,u6~=0
  Invalid : Subsystem  TreatAsAtomicUnit=on
  LV1 : Subsystem  AncestorBlock=tqr/TQR/Determine Torque Request/TorqueArbitrament/TorqueSmooth/Front First order filter input tau map and determination/VTQR_NORMALFEDUTs_c/LV1  TreatAsAtomicUnit=on
  LV2 : Subsystem  AncestorBlock=tqr/TQR/Determine Torque Request/TorqueArbitrament/TorqueSmooth/Front First order filter input tau map and determination/VTQR_NORMALFEDUTs_c/LV2  TreatAsAtomicUnit=on
  LV3 : Subsystem  AncestorBlock=tqr/TQR/Determine Torque Request/TorqueArbitrament/TorqueSmooth/Front First order filter input tau map and determination/VTQR_NORMALFEDUTs_c/LV3  TreatAsAtomicUnit=on
  LV4 : Subsystem  AncestorBlock=tqr/TQR/Determine Torque Request/TorqueArbitrament/TorqueSmooth/Front First order filter input tau map and determination/VTQR_NORMALFEDUTs_c/LV4  TreatAsAtomicUnit=on
  LV5 : Subsystem  AncestorBlock=tqr/TQR/Determine Torque Request/TorqueArbitrament/TorqueSmooth/Front First order filter input tau map and determination/VTQR_NORMALFEDUTs_c/LV5  TreatAsAtomicUnit=on
  Merge : Merge  Inputs=7
  OPD : Subsystem  AncestorBlock=tqr/TQR/Determine Torque Request/TorqueArbitrament/TorqueSmooth/Front First order filter input tau map and determination/VTQR_NORMALFEDUTs_c/OPD  TreatAsAtomicUnit=on
  VTQR_ECOFEDUTs_c : Outport
  wires:
  LV2/1(VTQR_EL2FEDUTs_c) -> Merge/2
  LV4/1(VTQR_EL4FEDUTs_c) -> Merge/4
  [VTQR_FEDUWhlTqReqSmoothDelay_Nm] -> LV1/1(VTQR_FEDUWhlTqReqSmoothDelay_Nm)
  Equal4/1 -> If/5
  [VTQD_TqTargetShaftSpd_rpm] -> LV3/2(VTQD_TqTargetShaftSpd_rpm)
  LV1/1(VTQR_EL1FEDUTsOrRegen_C) -> Merge/1
  Constant7/1 -> Equal1/2
  [VTQD_RegenMode_enum] -> Equal3/1
  VTQR_FEDUWhlTqReqSmoothDelay_Nm/1 -> [VTQR_FEDUWhlTqReqSmoothDelay_Nm]
  Constant11/1 -> Equal5/2
  [VTQD_TqTargetShaftSpd_rpm] -> OPD/2(VTQD_TqTargetShaftSpd_rpm)
  [VTQR_FEDUWhlTqReqSmoothDelay_Nm] -> OPD/1(VTQR_FEDUWhlTqReqSmoothDelay_Nm)
  Equal3/1 -> If/4
  LV3/1(VTQR_EL3FEDUTs_c) -> Merge/3
  Equal1/1 -> If/2
  VTQD_TqTargetShaftSpd_rpm/1 -> [VTQD_TqTargetShaftSpd_rpm]
  Equal2/1 -> If/3
  [VTQR_FEDUWhlTqReqSmoothDelay_Nm] -> LV3/1(VTQR_FEDUWhlTqReqSmoothDelay_Nm)
  VTQD_RegenMode_enum/1 -> [VTQD_RegenMode_enum]
  Equal/1 -> If/1
  [VTQD_TqTargetShaftSpd_rpm] -> LV4/2(VTQD_TqTargetShaftSpd_rpm)
  [VTQR_FEDUWhlTqReqSmoothDelay_Nm] -> LV4/1(VTQR_FEDUWhlTqReqSmoothDelay_Nm)
  OPD/1(VTQR_EOPDFEDUTs_c) -> Merge/6
  [VTQD_TqTargetShaftSpd_rpm] -> LV1/2(VTQD_TqTargetShaftSpd_rpm)
  Constant6/1 -> Equal/2
  [VTQD_TqTargetShaftSpd_rpm] -> LV2/2(VTQD_TqTargetShaftSpd_rpm)
  [VTQR_FEDUWhlTqReqSmoothDelay_Nm] -> LV2/1(VTQR_FEDUWhlTqReqSmoothDelay_Nm)
  [VTQD_RegenMode_enum] -> Equal2/1
  [VTQD_RegenMode_enum] -> Equal5/1
  Constant8/1 -> Equal2/2
  [VTQD_RegenMode_enum] -> Equal/1
  [VTQD_RegenMode_enum] -> Equal4/1
  Constant10/1 -> Equal4/2
  Constant9/1 -> Equal3/2
  [VTQD_TqTargetShaftSpd_rpm] -> LV5/2(VTQD_TqTargetShaftSpd_rpm)
  [VTQD_RegenMode_enum] -> Equal1/1
  LV5/1(VTQR_EL5FEDUTs_c) -> Merge/5
  Equal5/1 -> If/6
  [VTQR_FEDUWhlTqReqSmoothDelay_Nm] -> LV5/1(VTQR_FEDUWhlTqReqSmoothDelay_Nm)
  Merge/1 -> VTQR_ECOFEDUTs_c/1  "VTQR_ECOFEDUTs_c"
  VTQD_RollRegenEnable_flg/1 -> [VTQD_RollRegenEnable_flg]
  [VTQD_RollRegenEnable_flg] -> LV1/3(VTQD_RollRegenEnable_flg)
  [VTQD_RollRegenEnable_flg] -> Invalid/3(VTQD_RollRegenEnable_flg)
  [VTQD_TqTargetShaftSpd_rpm] -> Invalid/2(VTQD_TqTargetShaftSpd_rpm)
  [VTQR_FEDUWhlTqReqSmoothDelay_Nm] -> Invalid/1(VTQR_FEDUWhlTqReqSmoothDelay_Nm)
  If/1 -> LV1/Action
  If/2 -> LV2/Action
  If/3 -> LV3/Action
  If/4 -> LV4/Action
  If/5 -> LV5/Action
  If/6 -> OPD/Action
  If/7 -> Invalid/Action
  Invalid/1(VTQR_EL1FEDUTsOrRegen_C) -> Merge/7

== system tqr/TQR/Determine Torque Request/TorqueArbitrament/TorqueSmooth/Front First order filter input tau map and determination/VTQR_LHMFEDUTs_c ==
  VTQR_FEDUWhlTqReqSmoothDelay_Nm : Inport
  VTQD_TqTargetShaftSpd_rpm : Inport  Port=2
  Action Port : ActionPort  ActionPortLabel=if(u1~= 0)
  MTQR_LHMFEDUTs_Z_c : Lookup_n-D  BreakpointsForDimension1=ATQR_NL1FEDUTs_Y_Nm  BreakpointsForDimension2=ATQR_NL1FEDUTs_X_rpm  Table=MTQR_LHMFEDUTs_Z_c  ExtrapMethod=Clip  InternalRulePriority=Speed  RndMeth=Simplest  InputSameDT=on
      settings: InputPortMap=u0,u1
  VTQR_LHMFEDUTs_c : Outport
  wires:
  VTQR_FEDUWhlTqReqSmoothDelay_Nm/1 -> MTQR_LHMFEDUTs_Z_c/1
  VTQD_TqTargetShaftSpd_rpm/1 -> MTQR_LHMFEDUTs_Z_c/2
  MTQR_LHMFEDUTs_Z_c/1 -> VTQR_LHMFEDUTs_c/1  "VTQR_LHMFEDUTs_c"

== system tqr/TQR/Determine Torque Request/TorqueArbitrament/TorqueSmooth/Front First order filter input tau map and determination/VTQR_NORMALFEDUTs_c ==
  VTQR_FEDUWhlTqReqSmoothDelay_Nm : Inport
  VTQD_TqTargetShaftSpd_rpm : Inport  Port=2
  VTQD_RegenMode_enum : Inport  Port=3
  Action Port : ActionPort  ActionPortLabel=elseif(u4 ~= 0)
  Constant : Constant  Value=ENUM_REGENLEVEL_LV1
  Constant1 : Constant  Value=ENUM_REGENLEVEL_LV2
  Constant2 : Constant  Value=ENUM_REGENLEVEL_LV3
  Constant3 : Constant  Value=ENUM_REGENLEVEL_LV4
  Constant4 : Constant  Value=ENUM_REGENLEVEL_LV5
  Constant5 : Constant  Value=ENUM_REGENLEVEL_OPD
  Equal{,1..5} (6 alike) : RelationalOperator  Operator===  OutDataTypeStr=boolean  RndMeth=Simplest
  If : If  NumInputs=6  IfExpression=u1~= 0  ElseIfExpressions=u2 ~= 0, u3 ~= 0,u4 ~= 0,u5~=0,u6~=0
  Invalid : Subsystem  TreatAsAtomicUnit=on
  LV1 : Subsystem  TreatAsAtomicUnit=on
  LV2 : Subsystem  TreatAsAtomicUnit=on
  LV3 : Subsystem  TreatAsAtomicUnit=on
  LV4 : Subsystem  TreatAsAtomicUnit=on
  LV5 : Subsystem  TreatAsAtomicUnit=on
  Merge : Merge  Inputs=7
  OPD : Subsystem  AncestorBlock=tqr/TQR/Determine Torque Request/TorqueArbitrament/TorqueSmooth/Front First order filter input tau map and determination/VTQR_NORMALFEDUTs_c/LV5  TreatAsAtomicUnit=on
  VTQR_NORMALFEDUTs_c : Outport
  wires:
  VTQR_FEDUWhlTqReqSmoothDelay_Nm/1 -> [VTQR_FEDUWhlTqReqSmoothDelay_Nm]
  VTQD_TqTargetShaftSpd_rpm/1 -> [VTQD_TqTargetShaftSpd_rpm]
  VTQD_RegenMode_enum/1 -> [VTQD_RegenMode_enum]
  Constant/1 -> Equal/2
  [VTQD_RegenMode_enum] -> Equal/1
  Equal/1 -> If/1
  Equal1/1 -> If/2
  Constant1/1 -> Equal1/2
  [VTQD_RegenMode_enum] -> Equal1/1
  Equal2/1 -> If/3
  Constant2/1 -> Equal2/2
  [VTQD_RegenMode_enum] -> Equal2/1
  Equal3/1 -> If/4
  Constant3/1 -> Equal3/2
  [VTQD_RegenMode_enum] -> Equal3/1
  Equal4/1 -> If/5
  Constant4/1 -> Equal4/2
  [VTQD_RegenMode_enum] -> Equal4/1
  If/1 -> LV1/Action
  [VTQR_FEDUWhlTqReqSmoothDelay_Nm] -> LV1/1(VTQR_FEDUWhlTqReqSmoothDelay_Nm)
  [VTQD_TqTargetShaftSpd_rpm] -> LV1/2(VTQD_TqTargetShaftSpd_rpm)
  [VTQR_FEDUWhlTqReqSmoothDelay_Nm] -> LV2/1(VTQR_FEDUWhlTqReqSmoothDelay_Nm)
  [VTQD_TqTargetShaftSpd_rpm] -> LV2/2(VTQD_TqTargetShaftSpd_rpm)
  [VTQR_FEDUWhlTqReqSmoothDelay_Nm] -> LV3/1(VTQR_FEDUWhlTqReqSmoothDelay_Nm)
  [VTQD_TqTargetShaftSpd_rpm] -> LV3/2(VTQD_TqTargetShaftSpd_rpm)
  [VTQR_FEDUWhlTqReqSmoothDelay_Nm] -> LV4/1(VTQR_FEDUWhlTqReqSmoothDelay_Nm)
  [VTQD_TqTargetShaftSpd_rpm] -> LV4/2(VTQD_TqTargetShaftSpd_rpm)
  [VTQR_FEDUWhlTqReqSmoothDelay_Nm] -> LV5/1(VTQR_FEDUWhlTqReqSmoothDelay_Nm)
  [VTQD_TqTargetShaftSpd_rpm] -> LV5/2(VTQD_TqTargetShaftSpd_rpm)
  LV5/1(VTQR_NL5FEDUTs_c) -> Merge/5
  LV4/1(VTQR_NL4FEDUTs_c) -> Merge/4
  LV3/1(VTQR_NL3FEDUTs_c) -> Merge/3
  LV2/1(VTQR_NL2FEDUTs_c) -> Merge/2
  LV1/1(VTQR_NL1FEDUTs_c) -> Merge/1
  Equal5/1 -> If/6
  [VTQD_RegenMode_enum] -> Equal5/1
  Constant5/1 -> Equal5/2
  [VTQD_TqTargetShaftSpd_rpm] -> OPD/2(VTQD_TqTargetShaftSpd_rpm)
  [VTQR_FEDUWhlTqReqSmoothDelay_Nm] -> OPD/1(VTQR_FEDUWhlTqReqSmoothDelay_Nm)
  OPD/1(VTQR_NOPDFEDUTs_c) -> Merge/6
  Merge/1 -> VTQR_NORMALFEDUTs_c/1  "VTQR_NORMALFEDUTs_c"
  If/2 -> LV2/Action
  If/3 -> LV3/Action
  If/4 -> LV4/Action
  If/5 -> LV5/Action
  [VTQD_TqTargetShaftSpd_rpm] -> Invalid/2(VTQD_TqTargetShaftSpd_rpm)
  [VTQR_FEDUWhlTqReqSmoothDelay_Nm] -> Invalid/1(VTQR_FEDUWhlTqReqSmoothDelay_Nm)
  If/6 -> OPD/Action
  If/7 -> Invalid/Action
  Invalid/1(VTQR_NL1FEDUTs_c) -> Merge/7

== system tqr/TQR/Determine Torque Request/TorqueArbitrament/TorqueSmooth/Front First order filter input tau map and determination/VTQR_SNOWFEDUTs_c ==
  VTQR_FEDUWhlTqReqSmoothDelay_Nm : Inport
  VTQD_TqTargetShaftSpd_rpm : Inport  Port=2
  Action Port : ActionPort
  MTQR_SNOWFEDUTs_Z_c : Lookup_n-D  BreakpointsForDimension1=ATQR_NL1FEDUTs_Y_Nm  BreakpointsForDimension2=ATQR_NL1FEDUTs_X_rpm  Table=MTQR_SNOWFEDUTs_Z_c  ExtrapMethod=Clip  InternalRulePriority=Speed  RndMeth=Simplest  InputSameDT=on
      settings: InputPortMap=u0,u1
  VTQR_SNOWFEDUTs_c : Outport
  wires:
  VTQD_TqTargetShaftSpd_rpm/1 -> MTQR_SNOWFEDUTs_Z_c/2
  VTQR_FEDUWhlTqReqSmoothDelay_Nm/1 -> MTQR_SNOWFEDUTs_Z_c/1
  MTQR_SNOWFEDUTs_Z_c/1 -> VTQR_SNOWFEDUTs_c/1

== system tqr/TQR/Determine Torque Request/TorqueArbitrament/TorqueSmooth/Front First order filter input tau map and determination/VTQR_SPORTFEDUTs_c ==
  VTQR_FEDUWhlTqReqSmoothDelay_Nm : Inport
  VTQD_TqTargetShaftSpd_rpm : Inport  Port=2
  VTQD_RegenMode_enum : Inport  Port=3
  Action Port : ActionPort  ActionPortLabel=else
  Constant : Constant  Value=ENUM_REGENLEVEL_LV1
  Constant1 : Constant  Value=ENUM_REGENLEVEL_LV2
  Constant2 : Constant  Value=ENUM_REGENLEVEL_LV3
  Constant3 : Constant  Value=ENUM_REGENLEVEL_LV4
  Constant4 : Constant  Value=ENUM_REGENLEVEL_LV5
  Constant5 : Constant  Value=ENUM_REGENLEVEL_OPD
  Equal{,1..5} (6 alike) : RelationalOperator  Operator===  OutDataTypeStr=boolean  RndMeth=Simplest
  If : If  NumInputs=6  IfExpression=u1~= 0  ElseIfExpressions=u2 ~= 0, u3 ~= 0,u4 ~= 0,u5~=0,u6~=0
  Invalid : Subsystem  TreatAsAtomicUnit=on
  LV1 : Subsystem  AncestorBlock=tqr/TQR/Determine Torque Request/TorqueArbitrament/TorqueSmooth/Front First order filter input tau map and determination/VTQR_ECOFEDUTs_c/LV1  TreatAsAtomicUnit=on
  LV2 : Subsystem  AncestorBlock=tqr/TQR/Determine Torque Request/TorqueArbitrament/TorqueSmooth/Front First order filter input tau map and determination/VTQR_ECOFEDUTs_c/LV2  TreatAsAtomicUnit=on
  LV3 : Subsystem  AncestorBlock=tqr/TQR/Determine Torque Request/TorqueArbitrament/TorqueSmooth/Front First order filter input tau map and determination/VTQR_ECOFEDUTs_c/LV3  TreatAsAtomicUnit=on
  LV4 : Subsystem  AncestorBlock=tqr/TQR/Determine Torque Request/TorqueArbitrament/TorqueSmooth/Front First order filter input tau map and determination/VTQR_ECOFEDUTs_c/LV4  TreatAsAtomicUnit=on
  LV5 : Subsystem  AncestorBlock=tqr/TQR/Determine Torque Request/TorqueArbitrament/TorqueSmooth/Front First order filter input tau map and determination/VTQR_ECOFEDUTs_c/LV5  TreatAsAtomicUnit=on
  Merge : Merge  Inputs=7
  OPD : Subsystem  AncestorBlock=tqr/TQR/Determine Torque Request/TorqueArbitrament/TorqueSmooth/Front First order filter input tau map and determination/VTQR_ECOFEDUTs_c/OPD  TreatAsAtomicUnit=on
  VTQR_SPORTFEDUTs_c : Outport
  wires:
  [VTQD_TqTargetShaftSpd_rpm] -> LV4/2(VTQD_TqTargetShaftSpd_rpm)
  Equal/1 -> If/1
  OPD/1(VTQR_SOPDFEDUTs_c) -> Merge/6
  [VTQR_FEDUWhlTqReqSmoothDelay_Nm] -> LV4/1(VTQR_FEDUWhlTqReqSmoothDelay_Nm)
  [VTQR_FEDUWhlTqReqSmoothDelay_Nm] -> OPD/1(VTQR_FEDUWhlTqReqSmoothDelay_Nm)
  [VTQD_TqTargetShaftSpd_rpm] -> OPD/2(VTQD_TqTargetShaftSpd_rpm)
  VTQD_RegenMode_enum/1 -> [VTQD_RegenMode_enum]
  Equal3/1 -> If/4
  Equal1/1 -> If/2
  LV3/1(VTQR_SL3FEDUTs_c) -> Merge/3
  Equal2/1 -> If/3
  Constant5/1 -> Equal5/2
  Equal4/1 -> If/5
  LV1/1(VTQR_SL1FEDUTs_c) -> Merge/1
  [VTQD_TqTargetShaftSpd_rpm] -> LV3/2(VTQD_TqTargetShaftSpd_rpm)
  [VTQR_FEDUWhlTqReqSmoothDelay_Nm] -> LV1/1(VTQR_FEDUWhlTqReqSmoothDelay_Nm)
  VTQR_FEDUWhlTqReqSmoothDelay_Nm/1 -> [VTQR_FEDUWhlTqReqSmoothDelay_Nm]
  Constant1/1 -> Equal1/2
  LV4/1(VTQR_SL4FEDUTs_c) -> Merge/4
  [VTQD_RegenMode_enum] -> Equal3/1
  LV2/1(VTQR_SL2FEDUTs_c) -> Merge/2
  VTQD_TqTargetShaftSpd_rpm/1 -> [VTQD_TqTargetShaftSpd_rpm]
  [VTQR_FEDUWhlTqReqSmoothDelay_Nm] -> LV3/1(VTQR_FEDUWhlTqReqSmoothDelay_Nm)
  Constant3/1 -> Equal3/2
  [VTQD_TqTargetShaftSpd_rpm] -> LV5/2(VTQD_TqTargetShaftSpd_rpm)
  [VTQD_RegenMode_enum] -> Equal1/1
  [VTQR_FEDUWhlTqReqSmoothDelay_Nm] -> LV5/1(VTQR_FEDUWhlTqReqSmoothDelay_Nm)
  Equal5/1 -> If/6
  Constant4/1 -> Equal4/2
  LV5/1(VTQR_SL5FEDUTs_c) -> Merge/5
  Constant/1 -> Equal/2
  [VTQD_RegenMode_enum] -> Equal4/1
  Constant2/1 -> Equal2/2
  [VTQD_TqTargetShaftSpd_rpm] -> LV2/2(VTQD_TqTargetShaftSpd_rpm)
  [VTQD_TqTargetShaftSpd_rpm] -> LV1/2(VTQD_TqTargetShaftSpd_rpm)
  [VTQR_FEDUWhlTqReqSmoothDelay_Nm] -> LV2/1(VTQR_FEDUWhlTqReqSmoothDelay_Nm)
  [VTQD_RegenMode_enum] -> Equal/1
  [VTQD_RegenMode_enum] -> Equal5/1
  [VTQD_RegenMode_enum] -> Equal2/1
  Merge/1 -> VTQR_SPORTFEDUTs_c/1  "VTQR_SPORTFEDUTs_c"
  [VTQD_TqTargetShaftSpd_rpm] -> Invalid/2(VTQD_TqTargetShaftSpd_rpm)
  [VTQR_FEDUWhlTqReqSmoothDelay_Nm] -> Invalid/1(VTQR_FEDUWhlTqReqSmoothDelay_Nm)
  Invalid/1(VTQR_SL1FEDUTs_c) -> Merge/7
  If/1 -> LV1/Action
  If/2 -> LV2/Action
  If/3 -> LV3/Action
  If/4 -> LV4/Action
  If/5 -> LV5/Action
  If/6 -> OPD/Action
  If/7 -> Invalid/Action

== system tqr/TQR/Determine Torque Request/TorqueArbitrament/TorqueSmooth/Front First order filter input tau map and determination/VTQR_TCSFEDUTs_c ==
  VTQR_FEDUWhlTqReqSmoothDelay_Nm : Inport
  VTQD_TqTargetShaftSpd_rpm : Inport  Port=2
  Action Port : ActionPort
  MTQR_TCSFEDUTs_Z_c : Lookup_n-D  BreakpointsForDimension1=ATQR_NL1FEDUTs_Y_Nm  BreakpointsForDimension2=ATQR_NL1FEDUTs_X_rpm  Table=MTQR_TCSFEDUTs_Z_c  ExtrapMethod=Clip  InternalRulePriority=Speed  RndMeth=Simplest  InputSameDT=on
      settings: InputPortMap=u0,u1
  VTQR_TCSFEDUTs_c : Outport
  wires:
  VTQD_TqTargetShaftSpd_rpm/1 -> MTQR_TCSFEDUTs_Z_c/2
  VTQR_FEDUWhlTqReqSmoothDelay_Nm/1 -> MTQR_TCSFEDUTs_Z_c/1
  MTQR_TCSFEDUTs_Z_c/1 -> VTQR_TCSFEDUTs_c/1
